simulink model "eg_1_05_R2023a"  (R2023a)
settings: Solver=ode4  StartTime=0.0  StopTime=5  FixedStep=0.001  RelTol=1e-3  EnableMultiTasking=on
values from neighbouring files (symbols this model uses):
  k = 2    [eg_1_02b.m]    (also in eg_1_03b.m = - lqr(A,b,Q,R); eg_1_05.m; eg_1_06.m)
  kD1 = 2*M1*z1*wn1    (= 14)    [eg_1_05.m]
  kD2 = 2*M2*z2*wn2    (= 7)    [eg_1_05.m]
  kP1 = M1*wn1^2    (= 50)    [eg_1_05.m]
  kP2 = M2*wn2^2    (= 25)    [eg_1_05.m]
  M1 = 0.5    [eg_1_02b.m]    (also in eg_1_03b.m; eg_1_05.m = 2; eg_1_06.m = 2)
  M2 = 1    [eg_1_02b.m]    (also in eg_1_03b.m; eg_1_05.m; eg_1_06.m)
  mu = 1    [eg_1_02b.m]    (also in eg_1_03b.m; eg_1_05.m = 2; eg_1_06.m = 2)
  wn1 = 5    [eg_1_05.m]
  wn2 = 5    [eg_1_05.m]
  z1 = 0.7    [eg_1_05.m]
  z2 = 0.7    [eg_1_05.m]
settings Model: Creator=kawata  LastModifiedBy=kawata
settings SolverCC: AlgebraicLoopSolver=TrustRegion
settings DataIOCC: LimitDataPoints=on  SaveFormat=Array  SignalLoggingSaveFormat=ModelDataLogs  ReturnWorkspaceOutputs=off  SignalLoggingName=sigsOut
settings DebuggingCC: SaveWithParameterizedLinksMsg=none  UnderspecifiedInitializationDetection=Classic  MergeDetectMultiDrivingBlocksExec=none  SignalResolutionControl=TryResolveAllWithWarning  MultiTaskDSMMsg=warning  MultiTaskCondExecSysMsg=none  UnconnectedInputMsg=warning  UnconnectedOutputMsg=warning  UnconnectedLineMsg=warning  ArithmeticOperatorsInVariantConditions=warning
settings HardwareCC: TargetUnknown=on
settings ModelReferenceCC: EnableRefExpFcnMdlSchedulingChecks=on  PropagateSignalLabelsOutOfModel=off
settings SFSimCC: SimUseLocalCustomCode=off  CustomCodeUndefinedFunction=UseInterfaceOnly
settings RTWCC: RTWUseLocalCustomCode=off
settings GRTTargetCC: TargetFcnLib=ansi_tfl_tmw.mat  TargetLangStandard=C89/C90 (ANSI)  CombineOutputUpdateFcns=off  GRTInterface=on
settings ConfigComp: CovMetricSettings=dw  CovSaveCumulativeToWorkspaceVar=on  CovSaveSingleToWorkspaceVar=on  CovExternalEMLEnable=off

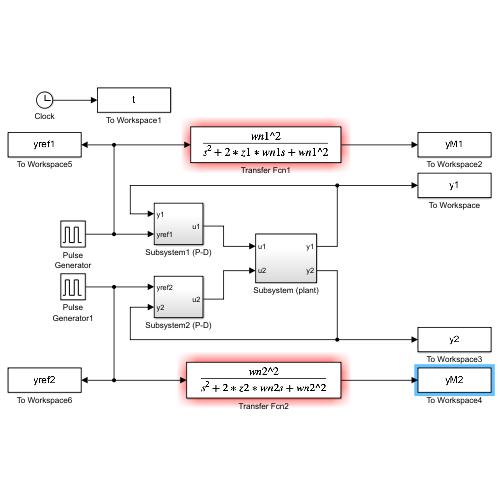
[thumbnail: Simulink's stored preview of the top-level diagram]
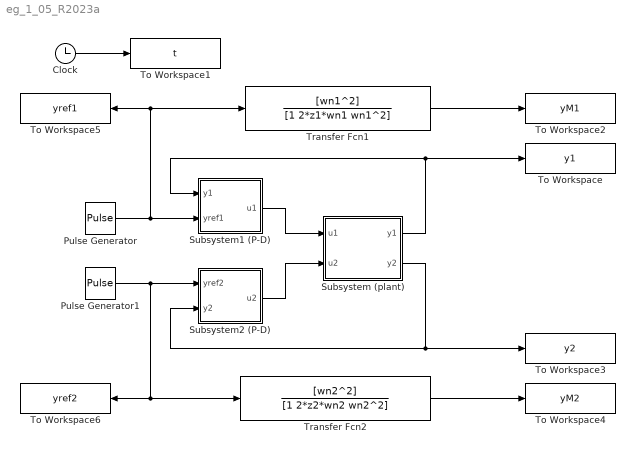
== system eg_1_05_R2023a ==
  Clock : Clock
  Pulse Generator : DiscretePulseGenerator  PulseType=Time based  Period=8  PulseWidth=50  PhaseDelay=2
  Pulse Generator1 : DiscretePulseGenerator  PulseType=Time based  Period=8  PulseWidth=50
  Subsystem (plant) : Subsystem
  Subsystem1 (P-D) : Subsystem
  Subsystem2 (P-D) : Subsystem
  To Workspace : ToWorkspace  VariableName=y1  SampleTime=-1
  To Workspace1 : ToWorkspace  VariableName=t  SampleTime=-1
  To Workspace2 : ToWorkspace  VariableName=yM1  SampleTime=-1
  To Workspace3 : ToWorkspace  VariableName=y2  SampleTime=-1
  To Workspace4 : ToWorkspace  VariableName=yM2  SampleTime=-1
  To Workspace5 : ToWorkspace  VariableName=yref1  SampleTime=-1
  To Workspace6 : ToWorkspace  VariableName=yref2  SampleTime=-1
  Transfer Fcn1 : TransferFcn  Numerator=[wn1^2]  Denominator=[1 2*z1*wn1 wn1^2]
  Transfer Fcn2 : TransferFcn  Numerator=[wn2^2]  Denominator=[1 2*z2*wn2 wn2^2]
  wires:
  Pulse Generator/1 -> Subsystem1 (P-D)/2(yref1), To Workspace5/1, Transfer Fcn1/1
  Clock/1 -> To Workspace1/1
  Pulse Generator1/1 -> Subsystem2 (P-D)/1(yref2), To Workspace6/1, Transfer Fcn2/1
  Subsystem1 (P-D)/1(u1) -> Subsystem (plant)/1(u1)
  Subsystem2 (P-D)/1(u2) -> Subsystem (plant)/2(u2)
  Subsystem (plant)/1(y1) -> To Workspace/1, Subsystem1 (P-D)/1(y1)
  Subsystem (plant)/2(y2) -> To Workspace3/1, Subsystem2 (P-D)/2(y2)
  Transfer Fcn1/1 -> To Workspace2/1
  Transfer Fcn2/1 -> To Workspace4/1

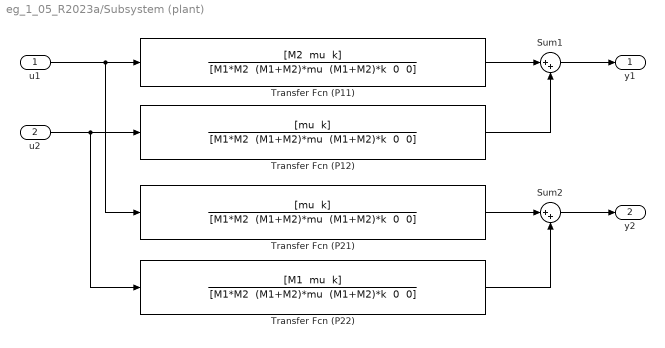
== system eg_1_05_R2023a/Subsystem (plant) ==
  u1 : Inport
  u2 : Inport  Port=2
  Sum1 : Sum  Inputs=|++  SaturateOnIntegerOverflow=on
  Sum2 : Sum  Inputs=|++  SaturateOnIntegerOverflow=on
  Transfer Fcn (P11) : TransferFcn  Numerator="[M2  mu  k]"  Denominator="[M1*M2  (M1+M2)*mu  (M1+M2)*k  0  0]"
  Transfer Fcn (P12) : TransferFcn  Numerator="[mu  k]"  Denominator="[M1*M2  (M1+M2)*mu  (M1+M2)*k  0  0]"
  Transfer Fcn (P21) : TransferFcn  Numerator="[mu  k]"  Denominator="[M1*M2  (M1+M2)*mu  (M1+M2)*k  0  0]"
  Transfer Fcn (P22) : TransferFcn  Numerator="[M1  mu  k]"  Denominator="[M1*M2  (M1+M2)*mu  (M1+M2)*k  0  0]"
  y1 : Outport  VectorParamsAs1DForOutWhenUnconnected=off
  y2 : Outport  Port=2  VectorParamsAs1DForOutWhenUnconnected=off
  wires:
  Transfer Fcn (P11)/1 -> Sum1/1
  Transfer Fcn (P12)/1 -> Sum1/2
  u1/1 -> Transfer Fcn (P11)/1, Transfer Fcn (P21)/1
  u2/1 -> Transfer Fcn (P12)/1, Transfer Fcn (P22)/1
  Transfer Fcn (P21)/1 -> Sum2/1
  Transfer Fcn (P22)/1 -> Sum2/2
  Sum1/1 -> y1/1
  Sum2/1 -> y2/1

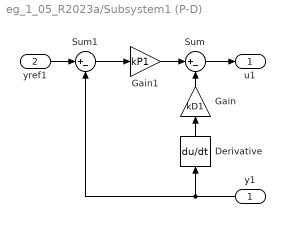
== system eg_1_05_R2023a/Subsystem1 (P-D) ==
  y1 : Inport
  yref1 : Inport  Port=2
  Derivative : Derivative
  Gain : Gain  Gain=kD1  SaturateOnIntegerOverflow=on  OutDataTypeStr=Inherit: Same as input  ParamDataTypeStr=Inherit: Same as input
  Gain1 : Gain  Gain=kP1  SaturateOnIntegerOverflow=on  OutDataTypeStr=Inherit: Same as input  ParamDataTypeStr=Inherit: Same as input
  Sum : Sum  Inputs=|+-  SaturateOnIntegerOverflow=on
  Sum1 : Sum  Inputs=|+-  SaturateOnIntegerOverflow=on
  u1 : Outport  VectorParamsAs1DForOutWhenUnconnected=off
  wires:
  Derivative/1 -> Gain/1
  Sum1/1 -> Gain1/1
  Gain1/1 -> Sum/1
  Gain/1 -> Sum/2
  Sum/1 -> u1/1
  yref1/1 -> Sum1/1
  y1/1 -> Sum1/2, Derivative/1

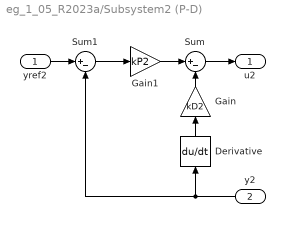
== system eg_1_05_R2023a/Subsystem2 (P-D) ==
  yref2 : Inport
  y2 : Inport  Port=2
  Derivative : Derivative
  Gain : Gain  Gain=kD2  SaturateOnIntegerOverflow=on  OutDataTypeStr=Inherit: Same as input  ParamDataTypeStr=Inherit: Same as input
  Gain1 : Gain  Gain=kP2  SaturateOnIntegerOverflow=on  OutDataTypeStr=Inherit: Same as input  ParamDataTypeStr=Inherit: Same as input
  Sum : Sum  Inputs=|+-  SaturateOnIntegerOverflow=on
  Sum1 : Sum  Inputs=|+-  SaturateOnIntegerOverflow=on
  u2 : Outport  VectorParamsAs1DForOutWhenUnconnected=off
  wires:
  y2/1 -> Derivative/1, Sum1/2
  yref2/1 -> Sum1/1
  Sum/1 -> u2/1
  Gain/1 -> Sum/2
  Gain1/1 -> Sum/1
  Sum1/1 -> Gain1/1
  Derivative/1 -> Gain/1
